simulink model "SimulacionMOASinLaplace"  (R2022a)
settings: Solver=VariableStepAuto  StartTime=0.0  StopTime=10  RelTol=1e-3
settings Model: Creator=Asus-PC  LastModifiedBy=Asus-PC

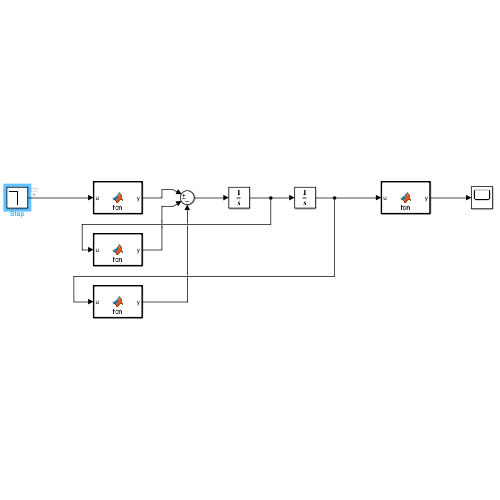
[thumbnail: Simulink's stored preview of the top-level diagram]
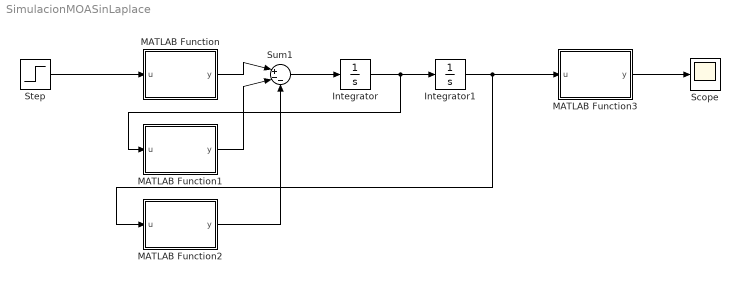
== system SimulacionMOASinLaplace ==
  Integrator : Integrator
  Integrator1 : Integrator
  MATLAB Function : MATLAB Function  TreatAsAtomicUnit=on
  MATLAB Function1 : MATLAB Function  TreatAsAtomicUnit=on
  MATLAB Function2 : MATLAB Function  TreatAsAtomicUnit=on
  MATLAB Function3 : MATLAB Function  TreatAsAtomicUnit=on
  Scope : Scope
  Step : Step  Time=0.01  Before=4080  After=0  SampleTime=0
  Sum1 : Sum  Inputs=|+--
  wires:
  Step/1 -> MATLAB Function/1(u)
  MATLAB Function/1(y) -> Sum1/1
  Sum1/1 -> Integrator/1
  MATLAB Function1/1(y) -> Sum1/2
  Integrator/1 -> MATLAB Function1/1(u), Integrator1/1
  MATLAB Function2/1(y) -> Sum1/3
  Integrator1/1 -> MATLAB Function3/1(u), MATLAB Function2/1(u)
  MATLAB Function3/1(y) -> Scope/1

== matlab function SimulacionMOASinLaplace/MATLAB Function ==
  data: u input; y output
function y = fcn(u)
y = u*(1/35.8);

== matlab function SimulacionMOASinLaplace/MATLAB Function2 ==
  data: u input; y output
function y = fcn(u)
y = u*(68600/35.8);

== matlab function SimulacionMOASinLaplace/MATLAB Function3 ==
  data: u input; y output
function y = fcn(u)
y = u;
fprintf('\n%f',y);

== matlab function SimulacionMOASinLaplace/MATLAB Function1 ==
  data: u input; y output
function y = fcn(u)
y = u*(100/35.8);
